simulink model "seven"  (R2020b)
settings: Solver=VariableStepAuto  StartTime=0.0  StopTime=10.0  RelTol=1e-3
undefined symbols (not defined in the file): a1, a2, b1, b2
settings Model: Creator=priyaD  LastModifiedBy=priyaD

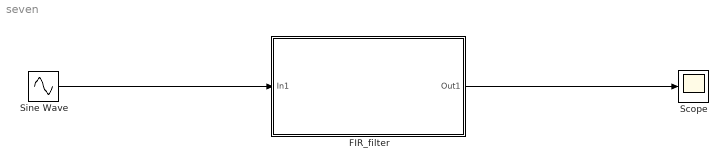
== system seven ==
  FIR_filter : Subsystem
  Scope : Scope
  Sine Wave : Sin  SampleTime=0
  wires:
  Sine Wave/1 -> FIR_filter/1(In1)
  FIR_filter/1(Out1) -> Scope/1

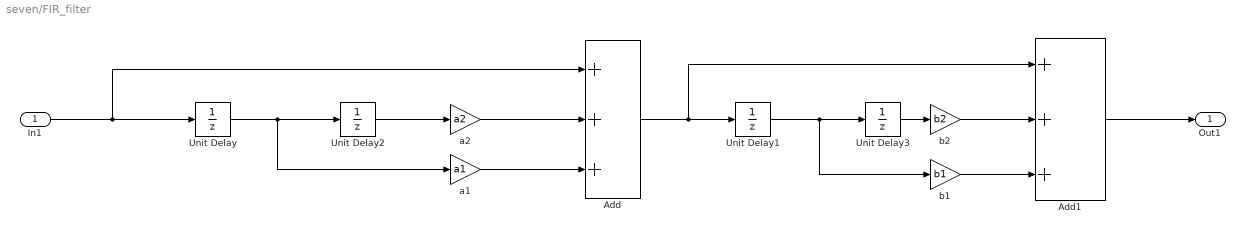
== system seven/FIR_filter ==
  In1 : Inport
  Add : Sum  Inputs=+++
  Add1 : Sum  Inputs=+++
  Unit Delay{,1..3} (4 alike) : UnitDelay  SampleTime=-1  HasFrameUpgradeWarning=on
  a1 : Gain  Gain=a1
  a2 : Gain  Gain=a2
  b1 : Gain  Gain=b1
  b2 : Gain  Gain=b2
  Out1 : Outport
  wires:
  b2/1 -> Add1/2
  Unit Delay3/1 -> b2/1
  Unit Delay1/1 -> b1/1, Unit Delay3/1
  a1/1 -> Add/3
  Add/1 -> Add1/1, Unit Delay1/1
  Unit Delay/1 -> a1/1, Unit Delay2/1
  b1/1 -> Add1/3
  Unit Delay2/1 -> a2/1
  In1/1 -> Add/1, Unit Delay/1
  a2/1 -> Add/2
  Add1/1 -> Out1/1
